simulink model "SecRwLtStHeightChk"  (R2018b)
settings: Solver=FixedStepDiscrete  StartTime=0.0  StopTime=10.0  FixedStep=0.01  RelTol=1e-3
undefined symbols (not defined in the file or in its folder): KeSMSeHeiCstTypeConfig_Val
libraries: simulink x3, HeightCalcLib x1
settings Model: Creator=sn2xws  LastModifiedBy=sn2xws
settings DataIOCC: SaveFormat=StructureWithTime
settings OptimizationCC: DefaultParameterBehavior=Inlined  EnhancedBackFolding=on  PassReuseOutputArgsAs=Individual arguments  ZeroExternalMemoryAtStartup=off  ZeroInternalMemoryAtStartup=off  OptimizeBlockOrder=speed  DifferentSizesBufferReuse=on  OptimizationCustomize=off
settings DebuggingCC: ParameterTunabilityLossMsg=error
settings ModelReferenceCC: ModelReferenceNumInstancesAllowed=Single
settings SFSimCC: MATLABDynamicMemAlloc=off
settings RTWCC: SystemTargetFile=autosar.tlc  GenCodeOnly=on  PackageGeneratedCodeAndArtifacts=on  PackageName=SecRwLtStHeightChk  TemplateMakefile=ert_default_tmf  Description=AUTOSAR  GenerateReport=on  IncludeHyperlinkInReport=on  LaunchReport=on  GenerateTraceInfo=on  GenerateTraceReport=on  GenerateTraceReportSl=on  GenerateTraceReportSf=on  GenerateTraceReportEml=on  GenerateCodeMetricsReport=on
settings CodeAppCC: ForceParamTrailComments=on  IgnoreCustomStorageClasses=off  OperatorAnnotations=on  SimulinkDataObjDesc=on  SFDataObjDesc=on  InsertBlockDesc=on
settings STFCustomTargetCC: TargetLangStandard=C99 (ISO)  MultiwordLength=256  ParMdlRefBuildCompliant=on  CompOptLevelCompliant=on  IncludeMdlTerminateFcn=off  CombineOutputUpdateFcns=on  SuppressErrorStatus=on  ERTCustomFileBanners=on  SupportNonFinite=off  SupportComplex=off  SupportContinuousTime=off  SupportNonInlinedSFcns=off  RemoveResetFunc=on  MATLABClassNameForMDSCustomization=Simulink.SoftwareTarget.ERTCustomization  AutosarCompliant=on  UseToolchainInfoCompliant=on  LookupTableObjectStructAxisOrder=2,1,3,4,...  LUTObjectStructOrderEvenSpacing=Size,Table,Breakpoints  SystemTargetFile=autosar.tlc
settings ERTTargetCC: TargetLangStandard=C99 (ISO)  ConcurrentExecutionCompliant=off  IncludeMdlTerminateFcn=off  SuppressErrorStatus=on  SupportNonFinite=off  SupportComplex=off  ModelStepFunctionPrototypeControlCompliant=off  CPPClassGenCompliant=off  AutosarCompliant=on  LookupTableObjectStructAxisOrder=2,1,3,4,...  LUTObjectStructOrderEvenSpacing=Size,Table,Breakpoints  InlinedParameterPlacement=NonHierarchical  ERTCustomFileTemplate=example_file_process.tlc  ERTFilePackagingFormat=Compact

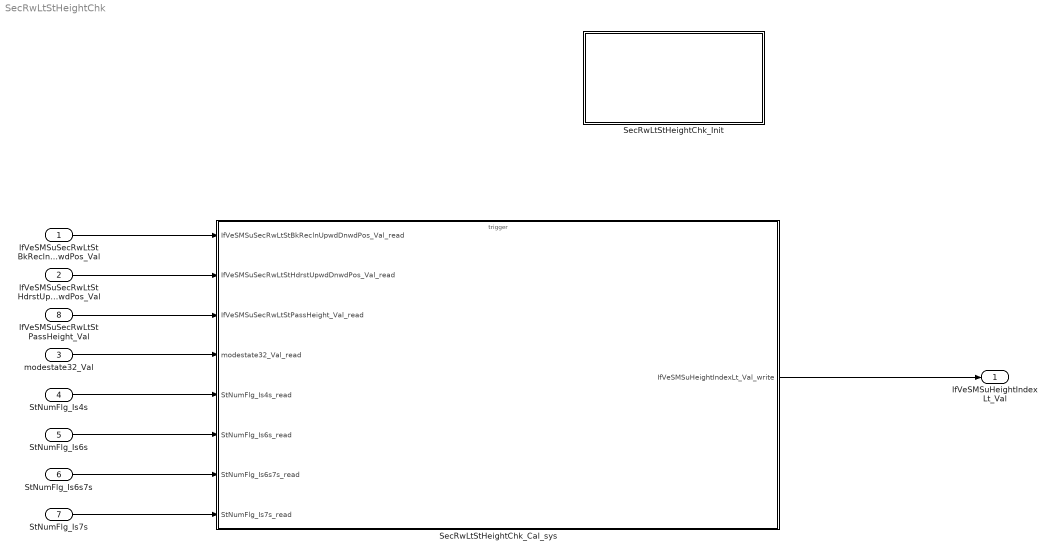
== system SecRwLtStHeightChk ==
  IfVeSMSuSecRwLtStBkReclnUpwdDnwdPos_Val : Inport  OutDataTypeStr=uint16  PortDimensions=1
  IfVeSMSuSecRwLtStHdrstUpwdDnwdPos_Val : Inport  Port=2  OutDataTypeStr=uint16  PortDimensions=1
  modestate32_Val : Inport  Port=3  OutDataTypeStr=uint32  PortDimensions=1
  StNumFlg_Is4s : Inport  Port=4  OutDataTypeStr=boolean  PortDimensions=1
  StNumFlg_Is6s : Inport  Port=5  OutDataTypeStr=boolean  PortDimensions=1
  StNumFlg_Is6s7s : Inport  Port=6  OutDataTypeStr=boolean  PortDimensions=1
  StNumFlg_Is7s : Inport  Port=7  OutDataTypeStr=boolean  PortDimensions=1
  IfVeSMSuSecRwLtStPassHeight_Val : Inport  Port=8  OutDataTypeStr=uint8  PortDimensions=1
  SecRwLtStHeightChk_Cal_sys : Subsystem
  SecRwLtStHeightChk_Init : Subsystem
  IfVeSMSuHeightIndexLt_Val : Outport  Description=|  OutDataTypeStr=uint8  PortDimensions=1
      | 0：under 160
      | 1：160
      | 2：165
      | 3：170
      | 4：175
      | 5：180
      | 6：over 180
  wires:
  IfVeSMSuSecRwLtStBkReclnUpwdDnwdPos_Val/1 -> SecRwLtStHeightChk_Cal_sys/1(IfVeSMSuSecRwLtStBkReclnUpwdDnwdPos_Val_read)
  IfVeSMSuSecRwLtStHdrstUpwdDnwdPos_Val/1 -> SecRwLtStHeightChk_Cal_sys/2(IfVeSMSuSecRwLtStHdrstUpwdDnwdPos_Val_read)
  modestate32_Val/1 -> SecRwLtStHeightChk_Cal_sys/4(modestate32_Val_read)
  StNumFlg_Is4s/1 -> SecRwLtStHeightChk_Cal_sys/5(StNumFlg_Is4s_read)
  StNumFlg_Is6s/1 -> SecRwLtStHeightChk_Cal_sys/6(StNumFlg_Is6s_read)
  StNumFlg_Is6s7s/1 -> SecRwLtStHeightChk_Cal_sys/7(StNumFlg_Is6s7s_read)
  StNumFlg_Is7s/1 -> SecRwLtStHeightChk_Cal_sys/8(StNumFlg_Is7s_read)
  IfVeSMSuSecRwLtStPassHeight_Val/1 -> SecRwLtStHeightChk_Cal_sys/3(IfVeSMSuSecRwLtStPassHeight_Val_read)
  SecRwLtStHeightChk_Cal_sys/1(IfVeSMSuHeightIndexLt_Val_write) -> IfVeSMSuHeightIndexLt_Val/1

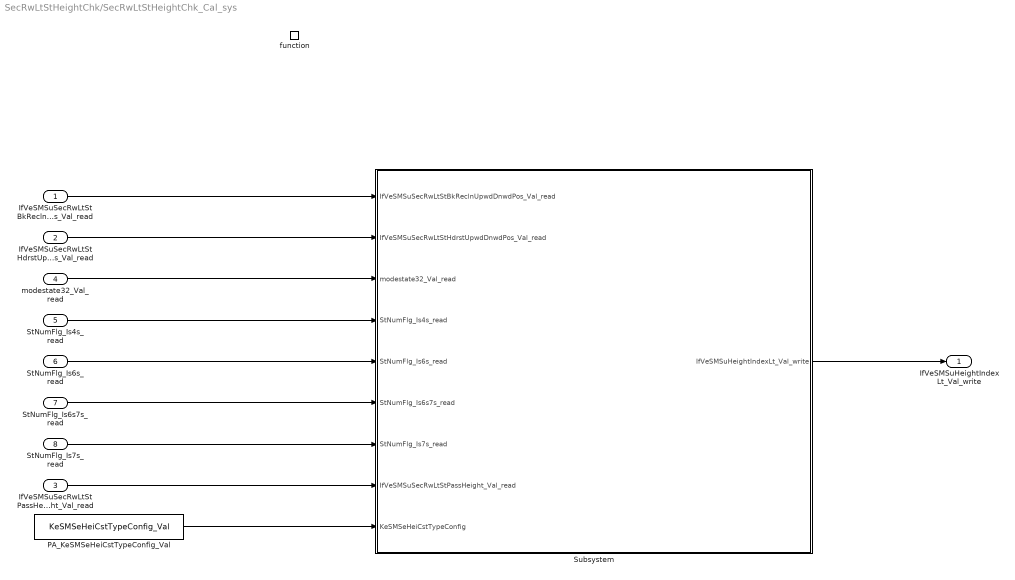
== system SecRwLtStHeightChk/SecRwLtStHeightChk_Cal_sys ==
  IfVeSMSuSecRwLtStBkReclnUpwdDnwdPos_Val_read : Inport
  IfVeSMSuSecRwLtStHdrstUpwdDnwdPos_Val_read : Inport  Port=2
  IfVeSMSuSecRwLtStPassHeight_Val_read : Inport  Port=3
  modestate32_Val_read : Inport  Port=4
  StNumFlg_Is4s_read : Inport  Port=5
  StNumFlg_Is6s_read : Inport  Port=6
  StNumFlg_Is6s7s_read : Inport  Port=7
  StNumFlg_Is7s_read : Inport  Port=8
  function : TriggerPort  TriggerType=function-call  IsSimulinkFunction=on  FunctionName=SecRwLtStHeightChk_Cal  VariantControl=(inherit)
  PA_KeSMSeHeiCstTypeConfig_Val : Constant  Value=KeSMSeHeiCstTypeConfig_Val
  Subsystem : Subsystem
  IfVeSMSuHeightIndexLt_Val_write : Outport
      settings: EnsureOutportIsVirtual=on
  wires:
  IfVeSMSuSecRwLtStBkReclnUpwdDnwdPos_Val_read/1 -> Subsystem/1(IfVeSMSuSecRwLtStBkReclnUpwdDnwdPos_Val_read)
  IfVeSMSuSecRwLtStHdrstUpwdDnwdPos_Val_read/1 -> Subsystem/2(IfVeSMSuSecRwLtStHdrstUpwdDnwdPos_Val_read)
  PA_KeSMSeHeiCstTypeConfig_Val/1 -> Subsystem/9(KeSMSeHeiCstTypeConfig)
  Subsystem/1(IfVeSMSuHeightIndexLt_Val_write) -> IfVeSMSuHeightIndexLt_Val_write/1
  IfVeSMSuSecRwLtStPassHeight_Val_read/1 -> Subsystem/8(IfVeSMSuSecRwLtStPassHeight_Val_read)
  modestate32_Val_read/1 -> Subsystem/3(modestate32_Val_read)
  StNumFlg_Is4s_read/1 -> Subsystem/4(StNumFlg_Is4s_read)
  StNumFlg_Is6s_read/1 -> Subsystem/5(StNumFlg_Is6s_read)
  StNumFlg_Is6s7s_read/1 -> Subsystem/6(StNumFlg_Is6s7s_read)
  StNumFlg_Is7s_read/1 -> Subsystem/7(StNumFlg_Is7s_read)

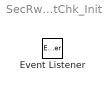
== system SecRwLtStHeightChk/SecRwLtStHeightChk_Init ==
  Event Listener : EventListener  EventName=reset

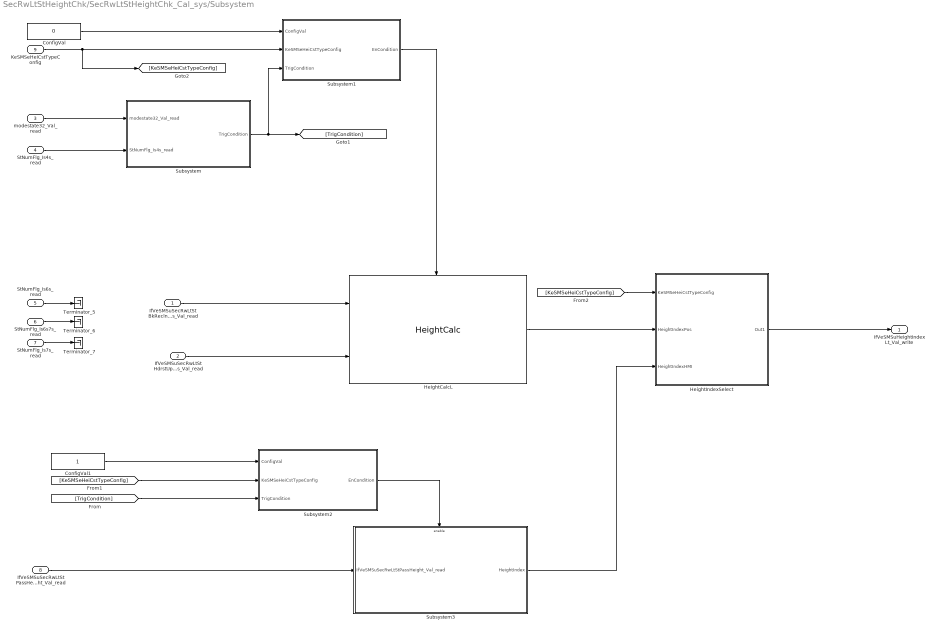
== system SecRwLtStHeightChk/SecRwLtStHeightChk_Cal_sys/Subsystem ==
  IfVeSMSuSecRwLtStBkReclnUpwdDnwdPos_Val_read : Inport
  IfVeSMSuSecRwLtStHdrstUpwdDnwdPos_Val_read : Inport  Port=2
  modestate32_Val_read : Inport  Port=3
  StNumFlg_Is4s_read : Inport  Port=4
  StNumFlg_Is6s_read : Inport  Port=5
  StNumFlg_Is6s7s_read : Inport  Port=6
  StNumFlg_Is7s_read : Inport  Port=7
  IfVeSMSuSecRwLtStPassHeight_Val_read : Inport  Port=8
  KeSMSeHeiCstTypeConfig : Inport  Port=9
  ConfigVal : Constant  Value=0  OutDataTypeStr=uint8
  ConfigVal1 : Constant  OutDataTypeStr=uint8
  HeightCalcL : HeightCalcLib/HeightCalc  SystemSampleTime=-1
  HeightIndexSelect : Subsystem
  Subsystem : Subsystem
  Subsystem1 : Subsystem
  Subsystem2 : Subsystem
  Subsystem3 : Subsystem
  Terminator_5 : Terminator
  Terminator_6 : Terminator
  Terminator_7 : Terminator
  IfVeSMSuHeightIndexLt_Val_write : Outport
      settings: EnsureOutportIsVirtual=on
  wires:
  StNumFlg_Is7s_read/1 -> Terminator_7/1
  IfVeSMSuSecRwLtStBkReclnUpwdDnwdPos_Val_read/1 -> HeightCalcL/1
  StNumFlg_Is6s7s_read/1 -> Terminator_6/1
  StNumFlg_Is6s_read/1 -> Terminator_5/1
  IfVeSMSuSecRwLtStHdrstUpwdDnwdPos_Val_read/1 -> HeightCalcL/2
  modestate32_Val_read/1 -> Subsystem/1(modestate32_Val_read)
  StNumFlg_Is4s_read/1 -> Subsystem/2(StNumFlg_Is4s_read)
  Subsystem/1(TrigCondition) -> [TrigCondition], Subsystem1/3(TrigCondition)
  KeSMSeHeiCstTypeConfig/1 -> [KeSMSeHeiCstTypeConfig], Subsystem1/2(KeSMSeHeiCstTypeConfig)
  Subsystem1/1(EnCondition) -> HeightCalcL/Enable
  ConfigVal/1 -> Subsystem1/1(ConfigVal)
  [TrigCondition] -> Subsystem2/3(TrigCondition)
  ConfigVal1/1 -> Subsystem2/1(ConfigVal)
  [KeSMSeHeiCstTypeConfig] -> Subsystem2/2(KeSMSeHeiCstTypeConfig)
  IfVeSMSuSecRwLtStPassHeight_Val_read/1 -> Subsystem3/1(IfVeSMSuSecRwLtStPassHeight_Val_read)
  Subsystem2/1(EnCondition) -> Subsystem3/Enable
  HeightCalcL/1 -> HeightIndexSelect/2(HeightIndexPos)
  Subsystem3/1(HeightIndex) -> HeightIndexSelect/3(HeightIndexHMI)
  HeightIndexSelect/1(Out1) -> IfVeSMSuHeightIndexLt_Val_write/1
  [KeSMSeHeiCstTypeConfig] -> HeightIndexSelect/1(KeSMSeHeiCstTypeConfig)

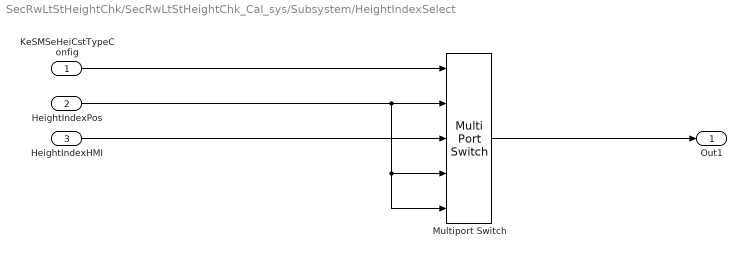
== system SecRwLtStHeightChk/SecRwLtStHeightChk_Cal_sys/Subsystem/HeightIndexSelect ==
  KeSMSeHeiCstTypeConfig : Inport
  HeightIndexPos : Inport  Port=2
  HeightIndexHMI : Inport  Port=3
  Multiport Switch : MultiPortSwitch  DataPortOrder=Zero-based contiguous  DataPortForDefault=Additional data port  DiagnosticForDefault=None  zeroidx=on
  Out1 : Outport
  wires:
  HeightIndexPos/1 -> Multiport Switch/5, Multiport Switch/4, Multiport Switch/2
  KeSMSeHeiCstTypeConfig/1 -> Multiport Switch/1
  Multiport Switch/1 -> Out1/1
  HeightIndexHMI/1 -> Multiport Switch/3

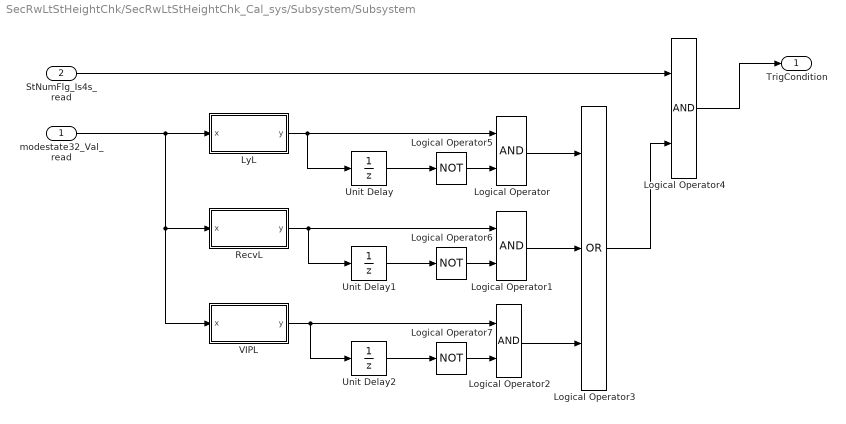
== system SecRwLtStHeightChk/SecRwLtStHeightChk_Cal_sys/Subsystem/Subsystem ==
  modestate32_Val_read : Inport
  StNumFlg_Is4s_read : Inport  Port=2
  Logical Operator{,1..2,4} (4 alike) : Logic  AllPortsSameDT=off  OutDataTypeStr=boolean
  Logical Operator3 : Logic  Operator=OR  Inputs=3  AllPortsSameDT=off  OutDataTypeStr=boolean
  Logical Operator5 : Logic  Operator=NOT  AllPortsSameDT=off  OutDataTypeStr=boolean
  Logical Operator6 : Logic  Operator=NOT  AllPortsSameDT=off  OutDataTypeStr=boolean
  Logical Operator7 : Logic  Operator=NOT  AllPortsSameDT=off  OutDataTypeStr=boolean
  LyL : Subsystem  mask(32 Bit Selector){BitNum=13}
      mask prompts: BitNum "Select Bit Number"
      mask help: Allows selection of a particular bit (0-31) out of a packed word up to 32 bits long. Output will be true if the bit number selected via the mask parameter is equal to one.
      mask TypeOptions BitNum: 0 | 1 | 2 | 3 | 4 | 5 | 6 | 7 | 8 | 9 | 10 | 11 | 12 | 13 | 14 | 15 | 16 | 17 | 18 | 19 | 20 | 21 | 22 | 23 | 24 | 25 | 26 | 27 | 28 | 29 | 30 | 31
      mask Display:
      | text(0.5, 0.8,'BIT','horizontalAlignment','center')
      | text(0.5, 0.5,'SELECTOR','horizontalAlignment','center')
      | text(0.5, 0.2,['-- Bit ',char(get_param(gcb,'BitNum')),' --'],'horizontalAlignment','center')
  RecvL : Subsystem  mask(32 Bit Selector){BitNum=10}
      mask prompts: BitNum "Select Bit Number"
      mask help: Allows selection of a particular bit (0-31) out of a packed word up to 32 bits long. Output will be true if the bit number selected via the mask parameter is equal to one.
      mask TypeOptions BitNum: 0 | 1 | 2 | 3 | 4 | 5 | 6 | 7 | 8 | 9 | 10 | 11 | 12 | 13 | 14 | 15 | 16 | 17 | 18 | 19 | 20 | 21 | 22 | 23 | 24 | 25 | 26 | 27 | 28 | 29 | 30 | 31
      mask Display:
      | text(0.5, 0.8,'BIT','horizontalAlignment','center')
      | text(0.5, 0.5,'SELECTOR','horizontalAlignment','center')
      | text(0.5, 0.2,['-- Bit ',char(get_param(gcb,'BitNum')),' --'],'horizontalAlignment','center')
  Unit Delay : UnitDelay  SampleTime=-1
  Unit Delay1 : UnitDelay  SampleTime=-1
  Unit Delay2 : UnitDelay  SampleTime=-1
  VIPL : Subsystem  mask(32 Bit Selector){BitNum=9}
      mask prompts: BitNum "Select Bit Number"
      mask help: Allows selection of a particular bit (0-31) out of a packed word up to 32 bits long. Output will be true if the bit number selected via the mask parameter is equal to one.
      mask TypeOptions BitNum: 0 | 1 | 2 | 3 | 4 | 5 | 6 | 7 | 8 | 9 | 10 | 11 | 12 | 13 | 14 | 15 | 16 | 17 | 18 | 19 | 20 | 21 | 22 | 23 | 24 | 25 | 26 | 27 | 28 | 29 | 30 | 31
      mask Display:
      | text(0.5, 0.8,'BIT','horizontalAlignment','center')
      | text(0.5, 0.5,'SELECTOR','horizontalAlignment','center')
      | text(0.5, 0.2,['-- Bit ',char(get_param(gcb,'BitNum')),' --'],'horizontalAlignment','center')
  TrigCondition : Outport
  wires:
  Logical Operator/1 -> Logical Operator3/1
  LyL/1(y) -> Unit Delay/1, Logical Operator/1
  RecvL/1(y) -> Unit Delay1/1, Logical Operator1/1
  Logical Operator1/1 -> Logical Operator3/2
  VIPL/1(y) -> Unit Delay2/1, Logical Operator2/1
  modestate32_Val_read/1 -> VIPL/1(x), RecvL/1(x), LyL/1(x)
  StNumFlg_Is4s_read/1 -> Logical Operator4/1
  Logical Operator2/1 -> Logical Operator3/3
  Logical Operator3/1 -> Logical Operator4/2
  Logical Operator4/1 -> TrigCondition/1
  Unit Delay/1 -> Logical Operator5/1
  Logical Operator5/1 -> Logical Operator/2
  Logical Operator6/1 -> Logical Operator1/2
  Unit Delay1/1 -> Logical Operator6/1
  Logical Operator7/1 -> Logical Operator2/2
  Unit Delay2/1 -> Logical Operator7/1

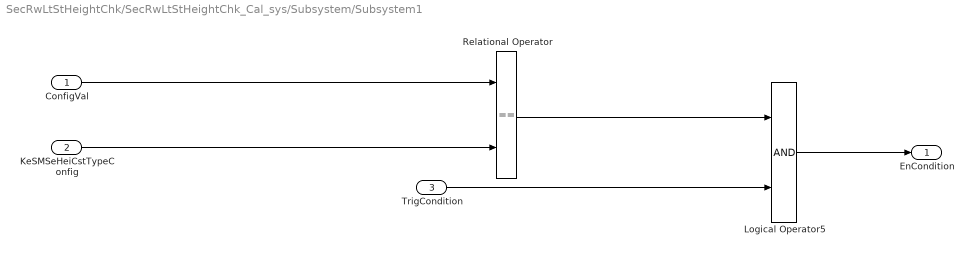
== system SecRwLtStHeightChk/SecRwLtStHeightChk_Cal_sys/Subsystem/Subsystem1 ==
  ConfigVal : Inport
  KeSMSeHeiCstTypeConfig : Inport  Port=2
  TrigCondition : Inport  Port=3
  Logical Operator5 : Logic  AllPortsSameDT=off  OutDataTypeStr=boolean
  Relational Operator : RelationalOperator  Operator===  OutDataTypeStr=boolean  RndMeth=Simplest
  EnCondition : Outport
  wires:
  Logical Operator5/1 -> EnCondition/1
  Relational Operator/1 -> Logical Operator5/1
  KeSMSeHeiCstTypeConfig/1 -> Relational Operator/2
  ConfigVal/1 -> Relational Operator/1
  TrigCondition/1 -> Logical Operator5/2

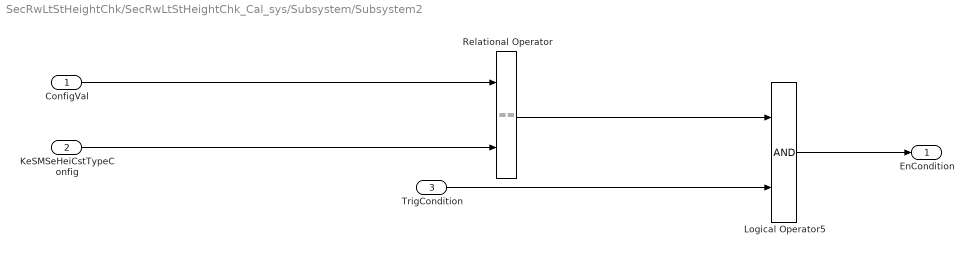
== system SecRwLtStHeightChk/SecRwLtStHeightChk_Cal_sys/Subsystem/Subsystem2 ==
  ConfigVal : Inport
  KeSMSeHeiCstTypeConfig : Inport  Port=2
  TrigCondition : Inport  Port=3
  Logical Operator5 : Logic  AllPortsSameDT=off  OutDataTypeStr=boolean
  Relational Operator : RelationalOperator  Operator===  OutDataTypeStr=boolean  RndMeth=Simplest
  EnCondition : Outport
  wires:
  TrigCondition/1 -> Logical Operator5/2
  ConfigVal/1 -> Relational Operator/1
  KeSMSeHeiCstTypeConfig/1 -> Relational Operator/2
  Relational Operator/1 -> Logical Operator5/1
  Logical Operator5/1 -> EnCondition/1

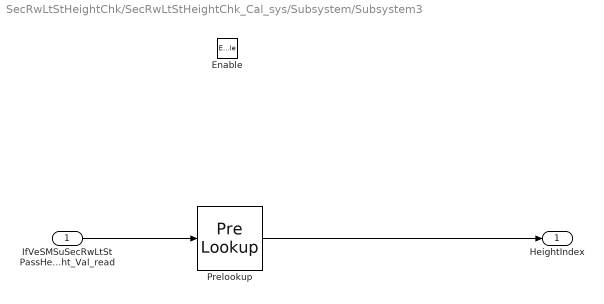
== system SecRwLtStHeightChk/SecRwLtStHeightChk_Cal_sys/Subsystem/Subsystem3 ==
  IfVeSMSuSecRwLtStPassHeight_Val_read : Inport
  Enable : EnablePort
  Prelookup : PreLookup  BreakpointsData=HeightIndexL  OutputSelection=Index only  RemoveProtectionInput=on  IndexDataTypeStr=uint8
  HeightIndex : Outport
  wires:
  IfVeSMSuSecRwLtStPassHeight_Val_read/1 -> Prelookup/1
  Prelookup/1 -> HeightIndex/1

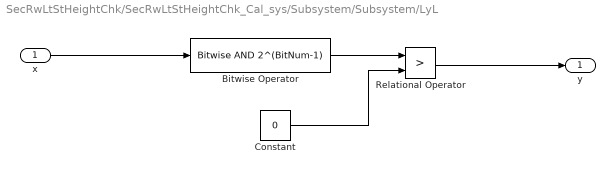
== system SecRwLtStHeightChk/SecRwLtStHeightChk_Cal_sys/Subsystem/Subsystem/LyL ==
  x : Inport
  Bitwise Operator : simulink/Logic and Bit Operations/Bitwise Operator  logicop=AND  UseBitMask=on  BitMask=2^(BitNum-1)  BitMaskRealWorld=Stored Integer
  Constant : Constant  Value=0  OutDataTypeStr=uint32
  Relational Operator : RelationalOperator  Operator=>  OutDataTypeStr=boolean  RndMeth=Simplest
  y : Outport
  wires:
  Relational Operator/1 -> y/1
  Constant/1 -> Relational Operator/2
  x/1 -> Bitwise Operator/1
  Bitwise Operator/1 -> Relational Operator/1

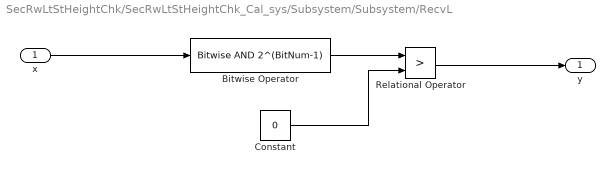
== system SecRwLtStHeightChk/SecRwLtStHeightChk_Cal_sys/Subsystem/Subsystem/RecvL ==
  x : Inport
  Bitwise Operator : simulink/Logic and Bit Operations/Bitwise Operator  logicop=AND  UseBitMask=on  BitMask=2^(BitNum-1)  BitMaskRealWorld=Stored Integer
  Constant : Constant  Value=0  OutDataTypeStr=uint32
  Relational Operator : RelationalOperator  Operator=>  OutDataTypeStr=boolean  RndMeth=Simplest
  y : Outport
  wires:
  Bitwise Operator/1 -> Relational Operator/1
  x/1 -> Bitwise Operator/1
  Constant/1 -> Relational Operator/2
  Relational Operator/1 -> y/1

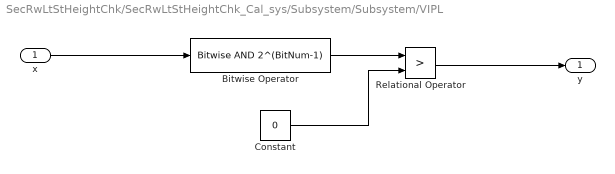
== system SecRwLtStHeightChk/SecRwLtStHeightChk_Cal_sys/Subsystem/Subsystem/VIPL ==
  x : Inport
  Bitwise Operator : simulink/Logic and Bit Operations/Bitwise Operator  logicop=AND  UseBitMask=on  BitMask=2^(BitNum-1)  BitMaskRealWorld=Stored Integer
  Constant : Constant  Value=0  OutDataTypeStr=uint32
  Relational Operator : RelationalOperator  Operator=>  OutDataTypeStr=boolean  RndMeth=Simplest
  y : Outport
  wires:
  Relational Operator/1 -> y/1
  Constant/1 -> Relational Operator/2
  x/1 -> Bitwise Operator/1
  Bitwise Operator/1 -> Relational Operator/1
